simulink model "untitled"  (R2022b)
settings: Solver=VariableStepAuto  StartTime=0.0  StopTime=10.0  RelTol=1e-3
values from neighbouring files (symbols this model uses):
  k = par(1)    [untitled.m]
  Tm = par(2)    [untitled.m]
  U_pr = 100    [untitled.m]
settings Model: Creator=redmi  LastModifiedBy=redmi

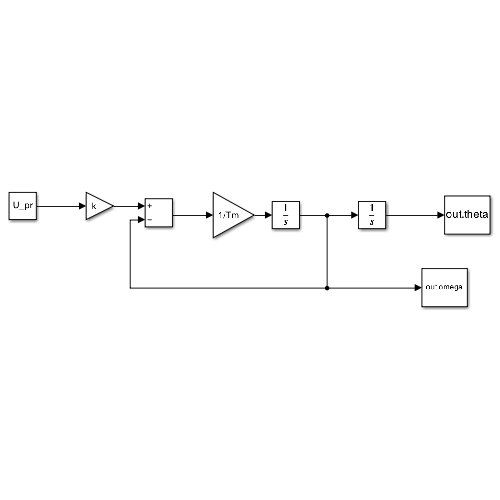
[thumbnail: Simulink's stored preview of the top-level diagram]
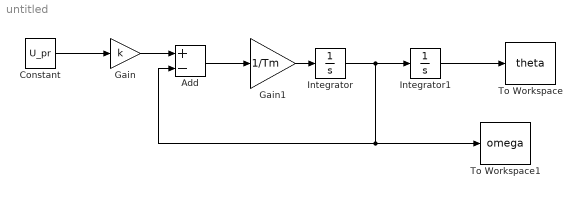
== system untitled ==
  Add : Sum  Inputs=+-
  Constant : Constant  Value=U_pr
  Gain : Gain  Gain=k
  Gain1 : Gain  Gain=1/Tm
  Integrator : Integrator
  Integrator1 : Integrator
  To Workspace : ToWorkspace  VariableName=theta  SampleTime=-1
      settings: Save2DSignal=2-D array (concatenate along first dimension)
  To Workspace1 : ToWorkspace  VariableName=omega  SampleTime=-1
      settings: Save2DSignal=2-D array (concatenate along first dimension)
  wires:
  Constant/1 -> Gain/1
  Gain/1 -> Add/1
  Add/1 -> Gain1/1
  Gain1/1 -> Integrator/1
  Integrator/1 -> Integrator1/1, To Workspace1/1, Add/2
  Integrator1/1 -> To Workspace/1
